simulink model "joytest"  (R2015a)
settings: Solver=ode45  StartTime=0.0  StopTime=inf  RelTol=1e-3
libraries: utility x1
settings Model: Creator=david.torres  LastModifiedBy=David
settings DebuggingCC: SolverPrmCheckMsg=warning

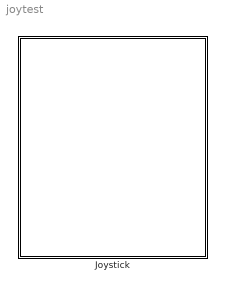
== system joytest ==
  Joystick : Subsystem

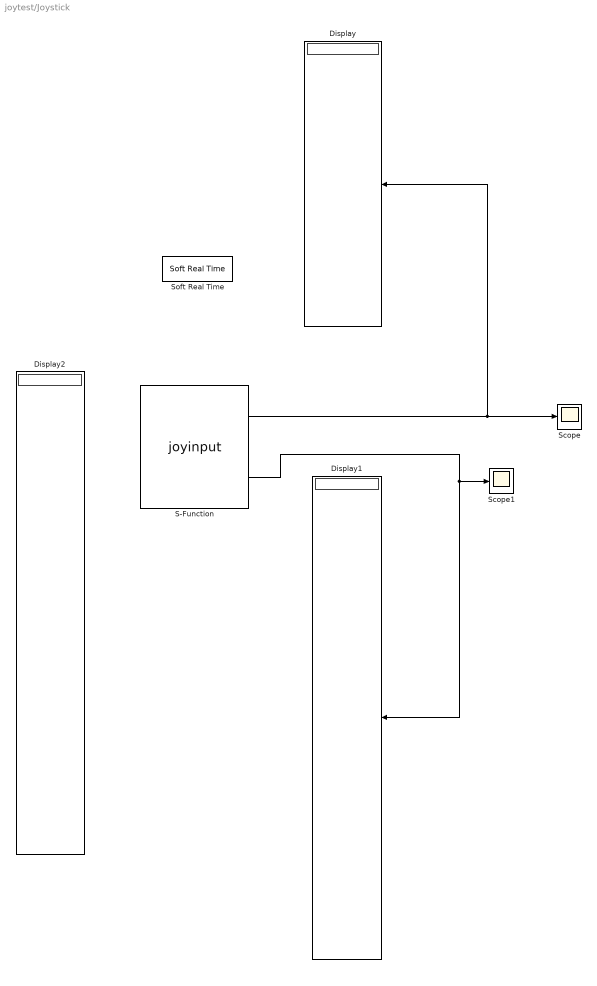
== system joytest/Joystick ==
  Display : Display
  Display1 : Display
  Display2 : Display
  S-Function : S-Function  FunctionName=joyinput  Parameters=joyid,adjustports,forcefeed  mask{joyid=1, adjustports=on, forcefeed=off}
      mask prompts: joyid "Joystick ID:"; adjustports "Adjust ports?"; forcefeed "Enable force"
      mask init:
      | label = 'image(imread(''joystickicon.png'')); port_label(''output'', 1, ''Axes''); port_label(''output'', 2, ''Buttons''); ';
      | porthandles = get_param(gcbh, 'PortHandles');
      | if numel(porthandles.Outport)>2
      |   label = [label 'port_label(''output'', 3, ''Point of View''); '];
      | end
      | if numel(porthandles.Inport)>0  label = [label 'port_label(''input'', 1, ''Force''); '];
      | end
      | set_param(gcbh, 'MaskDisplay', label);
      mask Help: helpview(vrmfunc('FnHelpTopic'), 'vr_joystickinput');
      mask Display: image(imread('joystickicon.png')); port_label('output', 1, 'Axes'); port_label('output', 2, 'Buttons');
  Scope : Scope
      settings: TimeRange=100  YMin=-1  YMax=1
  Scope1 : Scope
      settings: TimeRange=100
  Soft Real Time : utility/Soft Real Time  x=1
  wires:
  S-Function/1 -> Scope/1, Display/1
  S-Function/2 -> Display1/1, Scope1/1
  ? -> Display2/1
